simulink model "afe_abc_inv_3L_psm"  (R2025b)
settings: Solver=ode23tb  StartTime=0.0  StopTime=simlength  FixedStep=tc  MaxStep=tc
undefined symbols (not defined in the file or in its folder): Adrso, Amplitude_U, Amplitude_V, Amplitude_W, Aresd, b, Bresd, Cresd, Crso, CTRPIFF_CLIP_RELEASE, dead_time_AFE, dead_time_INV, deepNEGeta, deepNEGxi, deepPOSxi, emf_fb_p, emf_fb_p_ccaller_1, emf_fb_p_ccaller_2, emf_p, emf_p_ccaller_1, emf_p_ccaller_2, end_time_LVRT, fPWM_AFE, fPWM_INV, g0_161Hz, g0_500Hz, g1_161Hz, g1_500Hz, i_grid_neg_eta_lim, i_grid_neg_eta_red_lim, i_grid_neg_xi_lim, i_grid_neg_xi_red_lim, i_grid_pos_eta_lim, i_grid_pos_eta_red_lim, ibez, id_lim, ieta_neg_ref_lim, ieta_pos_ref_lim, Igrid_phase_normalization_factor, iq_lim, ixi_pos_ref_lim, Jm, k_frt_ref, kg, ki_afe, ki_i, ki_rc_neg_grid, ki_rc_pos_grid, ki_vs, ki_w, kp_afe, kp_i, kp_rc_neg_grid, kp_rc_pos_grid, kp_vs, kp_w, kw, l1, l2, Ld_norm ... (+48)
libraries: fl_lib x157, nesl_utility x86, cstblocks x14, simulink x13, single_phase_transformer_lib x3, threephase_inductor_lib x2, flexshaft_lib x1, pmsm_uvw_with_harmonics_lib x1
(part 6 of 11)

== system afe_abc_inv_3L_psm/afe_abc_inv_psm_mod1/inverter_control/current_ctrl/current_ctrl ==
  iq_ref : Inport
  MTPA : Subsystem
  Sqrt : Sqrt
  Square : Math  Operator=square
  Square1 : Math  Operator=square
  Sum : Sum  Inputs=|++
  To Workspace1 : ToWorkspace  VariableName=id_pu_sim  SampleTime=ts_inv
      settings: MaxDataPoints=Ns_inv
  To Workspace2 : ToWorkspace  VariableName=iq_pu_sim  SampleTime=ts_inv
      settings: MaxDataPoints=Ns_inv
  To Workspace3 : ToWorkspace  VariableName=id_ref_pu_sim  SampleTime=ts_inv
      settings: MaxDataPoints=Ns_inv
  To Workspace4 : ToWorkspace  VariableName=iq_ref_pu_sim  SampleTime=ts_inv
      settings: MaxDataPoints=Ns_inv
  To Workspace5 : ToWorkspace  VariableName=ud_pu_sim  SampleTime=ts_inv
      settings: MaxDataPoints=Ns_inv
  To Workspace6 : ToWorkspace  VariableName=uq_pu_sim  SampleTime=ts_inv
      settings: MaxDataPoints=Ns_inv
  To Workspace7 : ToWorkspace  VariableName=u_mot_pu_sim  SampleTime=ts_inv
      settings: MaxDataPoints=Ns_inv
  dq_pi_with_vector_antiwindup : Subsystem
  id_ref : Subsystem
      settings: PortSchema="{\"entries\":[{\"content\":{\"sides\":[{\"content\":{},\"type\":\"ConnectorPlacement.EquallySpacedRectSide\",\"uuid\":\"42af5d69-f0eb-42c6-9e03-28c1d0757323\"},{\"content\":{\"connectorIds\":[\"Out1\"],\"side\":\"RIGHT\"},\"type\":\"ConnectorPlacement.EquallySpacedRectSide\",\"uuid\":\"dd68a9f9-d15f-4e57-9d9e-130889a7b90c\"},{\"content\":{\"connectorIds\":[\"In1\"],\"side\":\"TOP\"},\"type\":\"ConnectorPlacement.EquallySpacedRectSide\",\"uuid\":\"68c797a2-8439-4b8d-8368-b7485adf0676\"}]},\"type\":\"ConnectorPlacement.EquallySpacedConnector\",\"uuid\":\"693c5f1c-0580-4626-8f13-b27865dfb3ac\"}],\"packageUris\":[\"http://schema.mathworks.com/mf0/Connector/R2020b\"],\"version\":\"1.0\"}"
  idref/id : Scope  NumInputPorts=2
      settings: SampleTime=tc  ActiveDisplayYMinimum=-0.65083541497562736  ActiveDisplayYMaximum=0.072495891063107235
  iqref/iq : Scope  NumInputPorts=2
      settings: SampleTime=tc  ActiveDisplayYMinimum=-1.1641617765003931  ActiveDisplayYMaximum=0.12935130850004364  DataLoggingVariableName=ScopeData2
  ud : Outport
  uq : Outport  Port=2
  tag scope: id_pu_ref=global, iq_pu_ref=global, u_mot_pu_sim=global, ud_pu_sim=global, uq_pu_sim=global
  wires:
  [iq_pu] -> To Workspace2/1, iqref/iq/2, dq_pi_with_vector_antiwindup/4(iq)  "iq"
  [id_pu] -> To Workspace1/1, idref/id/2, dq_pi_with_vector_antiwindup/2(id)  "id"
  MTPA/1(Id_ref_mtpa) -> id_ref/1(id_mtpa), [id_pu_ref]  "id_ref"
  iq_ref/1 -> MTPA/1(iq_ref), To Workspace4/1, iqref/iq/1, dq_pi_with_vector_antiwindup/3(iq_ref), [iq_pu_ref]  "iq_ref"
  dq_pi_with_vector_antiwindup/1(ctrl_d_u) -> To Workspace5/1, [ud_pu_sim], Square1/1, ud/1
  dq_pi_with_vector_antiwindup/2(ctrl_q_u) -> [uq_pu_sim], To Workspace6/1, Square/1, uq/1
  Square/1 -> Sum/1
  Sum/1 -> Sqrt/1
  Square1/1 -> Sum/2
  Sqrt/1 -> [u_mot_pu_sim], To Workspace7/1
  id_ref/1(id_ref) -> To Workspace3/1, dq_pi_with_vector_antiwindup/1(id_ref), idref/id/1  "id_ref"

== system afe_abc_inv_3L_psm/afe_abc_inv_psm_mod1/inverter_control/current_ctrl/current_transformation ==
  u : Inport
  v : Inport  Port=2
  w : Inport  Port=3
  To Workspace2 : ToWorkspace  VariableName=ialpha_pu_sim  SampleTime=ts_inv
      settings: MaxDataPoints=Ns_inv
  To Workspace3 : ToWorkspace  VariableName=ibeta_pu_sim  SampleTime=ts_inv
      settings: MaxDataPoints=Ns_inv
  alphabeta2dq : MATLAB Function  TreatAsAtomicUnit=on  SystemSampleTime=ts_inv
  uvw2alphabeta : MATLAB Function  TreatAsAtomicUnit=on  SystemSampleTime=ts_inv
  tag scope: ialpha_pu=global, ibeta_pu=global, id_pu=global, iq_pu=global
  wires:
  w/1 -> uvw2alphabeta/3(w)
  alphabeta2dq/2(q) -> [iq_pu]  "iq_pu"
  alphabeta2dq/1(d) -> [id_pu]  "id_pu"
  v/1 -> uvw2alphabeta/2(v)
  uvw2alphabeta/2(beta) -> To Workspace3/1, [ibeta_pu], alphabeta2dq/2(beta)  "ibeta_pu"
  uvw2alphabeta/1(alpha) -> To Workspace2/1, [ialpha_pu], alphabeta2dq/1(alpha)  "ialpha_pu"
  [theta_hat] -> alphabeta2dq/3(gamma)
  u/1 -> uvw2alphabeta/1(u)

== system afe_abc_inv_3L_psm/afe_abc_inv_psm_mod1/inverter_control/current_ctrl/sample_hold_normalization ==
  iu : Inport
  iv : Inport  Port=2
  iw : Inport  Port=3
  Gain : Gain  Gain=1/ibez
  Gain1 : Gain  Gain=1/ibez
  Gain2 : Gain  Gain=1/ibez
  Quantizer : Quantizer  QuantizationInterval=adc_quantization
  Quantizer1 : Quantizer  QuantizationInterval=adc_quantization
  Quantizer2 : Quantizer  QuantizationInterval=adc_quantization
  Unit Delay : UnitDelay  SampleTime=ts_inv  HasFrameUpgradeWarning=on
  Unit Delay1 : UnitDelay  SampleTime=ts_inv  HasFrameUpgradeWarning=on
  Unit Delay4 : UnitDelay  SampleTime=ts_inv  HasFrameUpgradeWarning=on
  Zero-Order Hold : ZeroOrderHold  SampleTime=ts_inv
  Zero-Order Hold1 : ZeroOrderHold  SampleTime=ts_inv
  Zero-Order Hold2 : ZeroOrderHold  SampleTime=ts_inv
  iu_pu : Outport
  iv_pu : Outport  Port=2
  iw_pu : Outport  Port=3
  wires:
  iu/1 -> Gain/1
  Zero-Order Hold1/1 -> Unit Delay1/1
  Zero-Order Hold2/1 -> Unit Delay4/1
  Zero-Order Hold/1 -> Unit Delay/1
  Unit Delay4/1 -> iw_pu/1
  Unit Delay1/1 -> iv_pu/1
  Unit Delay/1 -> iu_pu/1
  iw/1 -> Gain2/1
  iv/1 -> Gain1/1
  Gain2/1 -> Quantizer2/1
  Gain1/1 -> Quantizer1/1
  Gain/1 -> Quantizer/1
  Quantizer/1 -> Zero-Order Hold/1
  Quantizer1/1 -> Zero-Order Hold1/1
  Quantizer2/1 -> Zero-Order Hold2/1

== system afe_abc_inv_3L_psm/grid/grid_emulator/breaker/switch_1 ==
  Switch : fl_lib/Electrical/Electrical Elements/Switch  R_closed=Ron Ohm  G_open=1e-8 1/Ohm  Threshold=7.5  i_specify=off  i_priority=None  i=0 A  i_nominal_specify=off  i_nominal_value=1  i_nominal_unit=A  v_specify=off  v_priority=None  v=0 V  v_nominal_specify=off  v_nominal_value=1  v_nominal_unit=V
  snubber : fl_lib/Electrical/Electrical Elements/Capacitor  c=Csnubber F  r=Rsnubber Ohm  g=0 1/Ohm  i_specify=off  i_priority=None  i=0 A  i_nominal_specify=off  i_nominal_value=1  i_nominal_unit=A  v_specify=off  v_priority=None  v=0 V  v_nominal_specify=off  v_nominal_value=1  v_nominal_unit=V  vc_specify=off  vc_priority=High  vc=0 V  vc_nominal_specify=off  vc_nominal_value=1  vc_nominal_unit=V
  G : PMIOPort  Side=Left
  C : PMIOPort  Port=2  Side=Left
  E : PMIOPort  Port=3  Side=Right
  connections:
  Switch/RConn2 -- snubber/LConn1 -- C/RConn1
  Switch/RConn1 -- G/RConn1
  Switch/LConn1 -- snubber/RConn1 -- E/RConn1

== system afe_abc_inv_3L_psm/grid/grid_emulator/breaker/switch_2 ==
  Switch : fl_lib/Electrical/Electrical Elements/Switch  R_closed=Ron Ohm  G_open=1e-8 1/Ohm  Threshold=7.5  i_specify=off  i_priority=None  i=0 A  i_nominal_specify=off  i_nominal_value=1  i_nominal_unit=A  v_specify=off  v_priority=None  v=0 V  v_nominal_specify=off  v_nominal_value=1  v_nominal_unit=V
  snubber : fl_lib/Electrical/Electrical Elements/Capacitor  c=Csnubber F  r=Rsnubber Ohm  g=0 1/Ohm  i_specify=off  i_priority=None  i=0 A  i_nominal_specify=off  i_nominal_value=1  i_nominal_unit=A  v_specify=off  v_priority=None  v=0 V  v_nominal_specify=off  v_nominal_value=1  v_nominal_unit=V  vc_specify=off  vc_priority=High  vc=0 V  vc_nominal_specify=off  vc_nominal_value=1  vc_nominal_unit=V
  G : PMIOPort  Side=Left
  C : PMIOPort  Port=2  Side=Left
  E : PMIOPort  Port=3  Side=Right
  connections:
  snubber/RConn1 -- E/RConn1 -- Switch/LConn1
  Switch/RConn1 -- G/RConn1
  snubber/LConn1 -- C/RConn1 -- Switch/RConn2

== system afe_abc_inv_3L_psm/grid/grid_emulator/breaker/switch_3 ==
  Switch : fl_lib/Electrical/Electrical Elements/Switch  R_closed=Ron Ohm  G_open=1e-8 1/Ohm  Threshold=7.5  i_specify=off  i_priority=None  i=0 A  i_nominal_specify=off  i_nominal_value=1  i_nominal_unit=A  v_specify=off  v_priority=None  v=0 V  v_nominal_specify=off  v_nominal_value=1  v_nominal_unit=V
  snubber : fl_lib/Electrical/Electrical Elements/Capacitor  c=Csnubber F  r=Rsnubber Ohm  g=0 1/Ohm  i_specify=off  i_priority=None  i=0 A  i_nominal_specify=off  i_nominal_value=1  i_nominal_unit=A  v_specify=off  v_priority=None  v=0 V  v_nominal_specify=off  v_nominal_value=1  v_nominal_unit=V  vc_specify=off  vc_priority=High  vc=0 V  vc_nominal_specify=off  vc_nominal_value=1  vc_nominal_unit=V
  G : PMIOPort  Side=Left
  C : PMIOPort  Port=2  Side=Left
  E : PMIOPort  Port=3  Side=Right
  connections:
  Switch/RConn2 -- C/RConn1 -- snubber/LConn1
  Switch/RConn1 -- G/RConn1
  Switch/LConn1 -- E/RConn1 -- snubber/RConn1

== system afe_abc_inv_3L_psm/grid/grid_emulator/grid_emulator/phase_gen ==
  Constant4 : Constant  Value=omega_grid_emulator_nom
  Integrator : Integrator
  To Workspace7 : ToWorkspace  VariableName=gamma_grid_emulator_sim  SampleTime=ts_afe
      settings: MaxDataPoints=Ns_afe
  bounder1 : MATLAB Function  TreatAsAtomicUnit=on  SystemSampleTime=ts_afe
  grid_emu_phase : Outport  VectorParamsAs1DForOutWhenUnconnected=off
  tag scope: gamma_grid_emulator=global
  wires:
  bounder1/1(y) -> [gamma_grid_emulator], To Workspace7/1, grid_emu_phase/1  "grid_emu_phase"
  Constant4/1 -> Integrator/1
  Integrator/1 -> bounder1/1(u)

== system afe_abc_inv_3L_psm/grid/grid_emulator/grid_emulator/voltage_reference ==
  grid_emu_phase : Inport
  Vxi_p : Inport  Port=2
  Vxi_n : Inport  Port=3
  Veta_n : Inport  Port=4
  Constant2 : Constant  Value=0
  Sum1 : Sum  Inputs=|++
  Sum4 : Sum  Inputs=|++
  Variant Source : VariantSource  VariantControls={enable_frt_2 == 1, enable_frt_1 == 1}
  Variant Source1 : VariantSource  VariantControls={enable_frt_2 == 1, enable_frt_1 == 1}
  Variant Source2 : VariantSource  VariantControls={enable_frt_2 == 1, enable_frt_1 == 1}
  alphabeta2abc : MATLAB Function  TreatAsAtomicUnit=on  SystemSampleTime=ts_afe
  voltage_dource_with_frt : Subsystem
  xieta2alphabeta_neg : MATLAB Function  TreatAsAtomicUnit=on  SystemSampleTime=ts_afe
  xieta2alphabeta_pos : MATLAB Function  TreatAsAtomicUnit=on  SystemSampleTime=ts_afe
  V1_ref : Outport  VectorParamsAs1DForOutWhenUnconnected=off
  V2_ref : Outport  Port=2  VectorParamsAs1DForOutWhenUnconnected=off
  V3_ref : Outport  Port=3  VectorParamsAs1DForOutWhenUnconnected=off
  wires:
  xieta2alphabeta_pos/1(alpha) -> Sum1/1
  Sum1/1 -> alphabeta2abc/1(alpha)
  xieta2alphabeta_pos/2(beta) -> Sum4/1
  Sum4/1 -> alphabeta2abc/2(beta)
  xieta2alphabeta_neg/1(alpha) -> Sum1/2
  xieta2alphabeta_neg/2(beta) -> Sum4/2
  grid_emu_phase/1 -> voltage_dource_with_frt/1(gamma), xieta2alphabeta_neg/3(gamma), xieta2alphabeta_pos/3(gamma)
  Vxi_p/1 -> xieta2alphabeta_pos/1(xi)
  Constant2/1 -> xieta2alphabeta_pos/2(eta)
  Vxi_n/1 -> xieta2alphabeta_neg/1(xi)
  Veta_n/1 -> xieta2alphabeta_neg/2(eta)
  Variant Source/1 -> V1_ref/1
  alphabeta2abc/1(a) -> [V1_ref_xieta]
  alphabeta2abc/2(b) -> [V2_ref_xieta]
  alphabeta2abc/3(c) -> [V3_ref_xieta]
  voltage_dource_with_frt/3(vn_eta) -> [V3_ref_abc]
  voltage_dource_with_frt/2(vn_xi) -> [V2_ref_abc]
  voltage_dource_with_frt/1(vp_xi) -> [V1_ref_abc]
  [V1_ref_xieta] -> Variant Source/1
  [V1_ref_abc] -> Variant Source/2
  Variant Source1/1 -> V2_ref/1
  [V2_ref_xieta] -> Variant Source1/1
  [V2_ref_abc] -> Variant Source1/2
  Variant Source2/1 -> V3_ref/1
  [V3_ref_abc] -> Variant Source2/2
  [V3_ref_xieta] -> Variant Source2/1

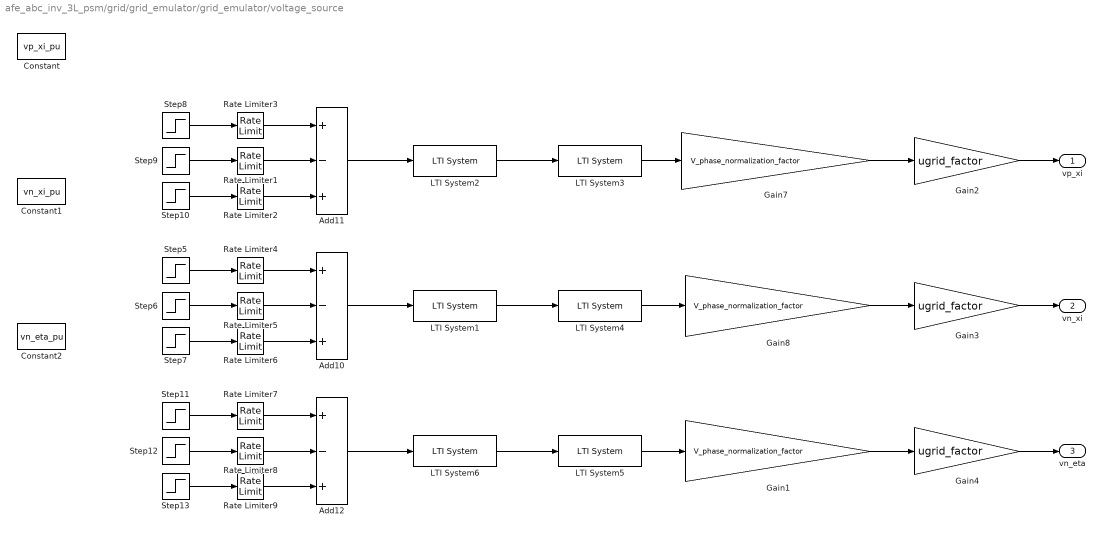
== system afe_abc_inv_3L_psm/grid/grid_emulator/grid_emulator/voltage_source ==
  Add10 : Sum  Inputs=+-+
  Add11 : Sum  Inputs=+-+
  Add12 : Sum  Inputs=+-+
  Constant : Constant  Value=vp_xi_pu
  Constant1 : Constant  Value=vn_xi_pu
  Constant2 : Constant  Value=vn_eta_pu
  Gain1 : Gain  Gain=V_phase_normalization_factor
  Gain2 : Gain  Gain=ugrid_factor
  Gain3 : Gain  Gain=ugrid_factor
  Gain4 : Gain  Gain=ugrid_factor
  Gain7 : Gain  Gain=V_phase_normalization_factor
  Gain8 : Gain  Gain=V_phase_normalization_factor
  LTI System1 : cstblocks/LTI System  sys=LVRT_flt_ss_c  IC=[0]  PadeOrder=0
  LTI System2 : cstblocks/LTI System  sys=LVRT_flt_ss_c  IC=[0]  PadeOrder=0
  LTI System3 : cstblocks/LTI System  sys=LVRT_flt_ss_c  IC=[]  PadeOrder=0
  LTI System4 : cstblocks/LTI System  sys=LVRT_flt_ss_c  IC=[]  PadeOrder=0
  LTI System5 : cstblocks/LTI System  sys=LVRT_flt_ss_c  IC=[]  PadeOrder=0
  LTI System6 : cstblocks/LTI System  sys=LVRT_flt_ss_c  IC=[0]  PadeOrder=0
  Rate Limiter{1..9} (9 alike) : RateLimiter  RisingSlewLimit=Vemu_ref_norm/t_ramp  FallingSlewLimit=-Vemu_ref_norm/t_ramp  SampleTimeMode=inherited
  Step10 : Step  Time=end_time_LVRT  After=vp_xi_pu*deepPOSxi  SampleTime=0
  Step11 : Step  Time=0  After=vn_eta_pu  SampleTime=0
  Step12 : Step  Time=start_time_LVRT  After=deepNEGeta  SampleTime=0
  Step13 : Step  Time=end_time_LVRT  After=deepNEGeta  SampleTime=0
  Step5 : Step  Time=0  After=vn_xi_pu  SampleTime=0
  Step6 : Step  Time=start_time_LVRT  After=deepNEGxi  SampleTime=0
  Step7 : Step  Time=end_time_LVRT  After=deepNEGxi  SampleTime=0
  Step8 : Step  Time=0  After=vp_xi_pu  SampleTime=0
  Step9 : Step  Time=start_time_LVRT  After=vp_xi_pu*deepPOSxi  SampleTime=0
  vp_xi : Outport  VectorParamsAs1DForOutWhenUnconnected=off
  vn_xi : Outport  Port=2  VectorParamsAs1DForOutWhenUnconnected=off
  vn_eta : Outport  Port=3  VectorParamsAs1DForOutWhenUnconnected=off
  wires:
  LTI System3/1 -> Gain7/1
  LTI System4/1 -> Gain8/1
  Gain7/1 -> Gain2/1
  Gain8/1 -> Gain3/1
  Gain1/1 -> Gain4/1
  LTI System5/1 -> Gain1/1
  Gain2/1 -> vp_xi/1
  Gain3/1 -> vn_xi/1
  Gain4/1 -> vn_eta/1
  LTI System6/1 -> LTI System5/1
  LTI System1/1 -> LTI System4/1
  LTI System2/1 -> LTI System3/1
  Rate Limiter2/1 -> Add11/3
  Add12/1 -> LTI System6/1
  Step7/1 -> Rate Limiter6/1
  Step6/1 -> Rate Limiter5/1
  Rate Limiter5/1 -> Add10/2
  Step5/1 -> Rate Limiter4/1
  Add11/1 -> LTI System2/1
  Rate Limiter7/1 -> Add12/1
  Step8/1 -> Rate Limiter3/1
  Step12/1 -> Rate Limiter8/1
  Step11/1 -> Rate Limiter7/1
  Rate Limiter1/1 -> Add11/2
  Step9/1 -> Rate Limiter1/1
  Rate Limiter3/1 -> Add11/1
  Rate Limiter8/1 -> Add12/2
  Rate Limiter9/1 -> Add12/3
  Rate Limiter4/1 -> Add10/1
  Rate Limiter6/1 -> Add10/3
  Step10/1 -> Rate Limiter2/1
  Add10/1 -> LTI System1/1
  Step13/1 -> Rate Limiter9/1

== system afe_abc_inv_3L_psm/grid/instantaneus_power/abc2alphabeta/abc2alphabeta ==
  a : Inport
  b : Inport  Port=2
  c : Inport  Port=3
  Gain1 : Gain  Gain=-1/2
  Gain11 : Gain  Gain=-1/2
  Gain2 : Gain  Gain=0
  Gain3 : Gain  Gain=sqrt(3)/2
  Gain4 : Gain  Gain=-sqrt(3)/2
  Gain8 : Gain  Gain=2/3
  Gain9 : Gain  Gain=2/3
  Sum : Sum  Inputs=+++
  Sum1 : Sum  Inputs=+++
  "alpha " : Outport  VectorParamsAs1DForOutWhenUnconnected=off
  "beta " : Outport  Port=2  VectorParamsAs1DForOutWhenUnconnected=off
  wires:
  Gain11/1 -> Sum/2
  Gain1/1 -> Sum/3
  Gain9/1 -> "beta "/1
  Gain8/1 -> "alpha "/1
  Gain2/1 -> Sum1/1
  Gain3/1 -> Sum1/2
  Gain4/1 -> Sum1/3
  a/1 -> Gain2/1, Sum/1
  c/1 -> Gain4/1, Gain1/1
  b/1 -> Gain3/1, Gain11/1
  Sum/1 -> Gain8/1
  Sum1/1 -> Gain9/1

== system afe_abc_inv_3L_psm/grid/instantaneus_power/abc2alphabeta /abc->alphabeta ==
  a : Inport
  b : Inport  Port=2
  c : Inport  Port=3
  Gain1 : Gain  Gain=-1/2
  Gain11 : Gain  Gain=-1/2
  Gain2 : Gain  Gain=0
  Gain3 : Gain  Gain=sqrt(3)/2
  Gain4 : Gain  Gain=-sqrt(3)/2
  Gain8 : Gain  Gain=2/3
  Gain9 : Gain  Gain=2/3
  Sum : Sum  Inputs=+++
  Sum1 : Sum  Inputs=+++
  "alpha " : Outport  VectorParamsAs1DForOutWhenUnconnected=off
  "beta " : Outport  Port=2  VectorParamsAs1DForOutWhenUnconnected=off
  wires:
  Sum1/1 -> Gain9/1
  Sum/1 -> Gain8/1
  b/1 -> Gain11/1, Gain3/1
  c/1 -> Gain1/1, Gain4/1
  a/1 -> Sum/1, Gain2/1
  Gain4/1 -> Sum1/3
  Gain3/1 -> Sum1/2
  Gain2/1 -> Sum1/1
  Gain8/1 -> "alpha "/1
  Gain9/1 -> "beta "/1
  Gain1/1 -> Sum/3
  Gain11/1 -> Sum/2

== system afe_abc_inv_3L_psm/afe_abc_inv_psm_mod1/afe/sv_pwm/modulator1/PWM generator u ==
  m : Inport
  phase : Inport  Port=2
  Bus Creator : BusCreator  Inputs=4
  Constant : Constant
  Gain : Gain  Gain=2
  Sum : Sum  Inputs=|+-
  carry_p : Subsystem
  modulator_n1 : Subsystem
  modulator_p1 : Subsystem
  mu : Outport
  wires:
  phase/1 -> carry_p/1(phase)
  carry_p/1(trp) -> modulator_n1/1(tr), modulator_p1/1(tr)  "trp"
  modulator_p1/1(m1) -> [m1]
  modulator_p1/2(m3) -> [m3]
  modulator_n1/1(m2) -> [m2]
  modulator_n1/2(m4) -> [m4]
  [m1] -> Bus Creator/1  "m1u"
  [m2] -> Bus Creator/2  "m2u"
  [m3] -> Bus Creator/3  "m3u"
  [m4] -> Bus Creator/4  "m4u"
  Bus Creator/1 -> mu/1  "p"
  m/1 -> Gain/1
  Gain/1 -> Sum/1
  Constant/1 -> Sum/2
  Sum/1 -> modulator_p1/2(m_index), modulator_n1/2(m_index)

== system afe_abc_inv_3L_psm/afe_abc_inv_psm_mod1/afe/sv_pwm/modulator1/PWM generator v ==
  m : Inport
  phase : Inport  Port=2
  Bus Creator : BusCreator  Inputs=4
  Constant : Constant
  Gain : Gain  Gain=2
  Sum : Sum  Inputs=|+-
  carry_p : Subsystem
  modulator_n1 : Subsystem
  modulator_p1 : Subsystem
  mv : Outport
  wires:
  Sum/1 -> modulator_n1/2(m_index), modulator_p1/2(m_index)
  Constant/1 -> Sum/2
  Gain/1 -> Sum/1
  m/1 -> Gain/1
  Bus Creator/1 -> mv/1  "p"
  [m4] -> Bus Creator/4  "m4v"
  [m3] -> Bus Creator/3  "m3v"
  [m2] -> Bus Creator/2  "m2v"
  [m1] -> Bus Creator/1  "m1v"
  modulator_n1/2(m4) -> [m4]
  modulator_n1/1(m2) -> [m2]
  modulator_p1/2(m3) -> [m3]
  modulator_p1/1(m1) -> [m1]
  carry_p/1(trp) -> modulator_p1/1(tr), modulator_n1/1(tr)  "trp"
  phase/1 -> carry_p/1(phase)

== system afe_abc_inv_3L_psm/afe_abc_inv_psm_mod1/afe/sv_pwm/modulator1/PWM generator w ==
  m : Inport
  phase : Inport  Port=2
  Bus Creator : BusCreator  Inputs=4
  Constant : Constant
  Gain : Gain  Gain=2
  Sum : Sum  Inputs=|+-
  carry_p : Subsystem
  modulator_n1 : Subsystem
  modulator_p1 : Subsystem
  mw : Outport
  wires:
  phase/1 -> carry_p/1(phase)
  carry_p/1(trp) -> modulator_n1/1(tr), modulator_p1/1(tr)  "trp"
  modulator_p1/1(m1) -> [m1]
  modulator_p1/2(m3) -> [m3]
  modulator_n1/1(m2) -> [m2]
  modulator_n1/2(m4) -> [m4]
  [m1] -> Bus Creator/1  "m1w"
  [m2] -> Bus Creator/2  "m2w"
  [m3] -> Bus Creator/3  "m3w"
  [m4] -> Bus Creator/4  "m4w"
  Bus Creator/1 -> mw/1  "p"
  m/1 -> Gain/1
  Gain/1 -> Sum/1
  Constant/1 -> Sum/2
  Sum/1 -> modulator_p1/2(m_index), modulator_n1/2(m_index)

== system afe_abc_inv_3L_psm/afe_abc_inv_psm_mod1/afe_control/current_ctrl/Inner Loop Current Control/Current-Control, Phase a ==
  In1 : Inport
  In2 : Inport  Port=2
  Add : Sum
  Cresd./Tcontrol new1 : Gain  Gain=Cresd  Multiplication=Matrix(K*u)
  Gain : Gain  Gain=kp_afe
  Gain1 : Gain  Gain=ki_afe
  Gain2 : Gain  Gain=Bresd  Multiplication=Matrix(K*u)
  Gain3 : Gain  Gain=Aresd  Multiplication=Matrix(K*u)
  Gain4 : Gain  Gain=1/ts_afe
  Gain5 : Gain  Gain=ts_afe
  Sum : Sum  Inputs=|+-
  Sum2 : Sum  Inputs=|++  SaturateOnIntegerOverflow=on
  Unit Delay : UnitDelay  InitialCondition=[0 0]  SampleTime=ts_afe  HasFrameUpgradeWarning=on
  Out1 : Outport
  wires:
  In1/1 -> Sum/1  "isa_ref"
  In2/1 -> Sum/2  "isa"
  Add/1 -> Out1/1  "v_a"
  Sum/1 -> Gain1/1, Gain/1
  Gain/1 -> Add/1
  Gain1/1 -> Gain2/1  "u(k)"
  Gain2/1 -> Gain5/1
  Gain5/1 -> Sum2/1
  Unit Delay/1 -> Gain3/1, Cresd./Tcontrol new1/1  "x(k)"
  Sum2/1 -> Unit Delay/1  "x(k+1)"
  Gain3/1 -> Sum2/2
  Cresd./Tcontrol new1/1 -> Gain4/1  "y(k)"
  Gain4/1 -> Add/2

== system afe_abc_inv_3L_psm/afe_abc_inv_psm_mod1/afe_control/current_ctrl/Inner Loop Current Control/Current-Control, Phase b ==
  In1 : Inport
  In2 : Inport  Port=2
  Add : Sum
  Cresd./Tcontrol new1 : Gain  Gain=Cresd  Multiplication=Matrix(K*u)
  Gain : Gain  Gain=kp_afe
  Gain1 : Gain  Gain=ki_afe
  Gain2 : Gain  Gain=Bresd  Multiplication=Matrix(K*u)
  Gain3 : Gain  Gain=Aresd  Multiplication=Matrix(K*u)
  Gain4 : Gain  Gain=1/ts_afe
  Gain5 : Gain  Gain=ts_afe
  Sum : Sum  Inputs=|+-
  Sum2 : Sum  Inputs=|++  SaturateOnIntegerOverflow=on
  Unit Delay : UnitDelay  InitialCondition=[0 0]  SampleTime=ts_afe  HasFrameUpgradeWarning=on
  Out1 : Outport
  wires:
  Cresd./Tcontrol new1/1 -> Gain4/1  "y(k)"
  Gain3/1 -> Sum2/2
  Sum2/1 -> Unit Delay/1  "x(k+1)"
  Unit Delay/1 -> Cresd./Tcontrol new1/1, Gain3/1  "x(k)"
  Gain5/1 -> Sum2/1
  Gain2/1 -> Gain5/1
  Gain1/1 -> Gain2/1  "u(k)"
  Gain/1 -> Add/1
  Sum/1 -> Gain/1, Gain1/1
  Add/1 -> Out1/1  "v_a"
  In2/1 -> Sum/2  "isb"
  In1/1 -> Sum/1  "isb_ref"
  Gain4/1 -> Add/2

== system afe_abc_inv_3L_psm/afe_abc_inv_psm_mod1/afe_control/current_ctrl/Inner Loop Current Control/Current-Control, Phase c ==
  In1 : Inport
  In2 : Inport  Port=2
  Add : Sum
  Cresd./Tcontrol new1 : Gain  Gain=Cresd  Multiplication=Matrix(K*u)
  Gain : Gain  Gain=kp_afe
  Gain1 : Gain  Gain=ki_afe
  Gain2 : Gain  Gain=Bresd  Multiplication=Matrix(K*u)
  Gain3 : Gain  Gain=Aresd  Multiplication=Matrix(K*u)
  Gain4 : Gain  Gain=1/ts_afe
  Gain5 : Gain  Gain=ts_afe
  Sum : Sum  Inputs=|+-
  Sum2 : Sum  Inputs=|++  SaturateOnIntegerOverflow=on
  Unit Delay : UnitDelay  InitialCondition=[0 0]  SampleTime=ts_afe  HasFrameUpgradeWarning=on
  Out1 : Outport
  wires:
  In1/1 -> Sum/1  "isc_ref"
  In2/1 -> Sum/2  "isc"
  Add/1 -> Out1/1  "v_a"
  Sum/1 -> Gain1/1, Gain/1
  Gain/1 -> Add/1
  Gain1/1 -> Gain2/1  "u(k)"
  Gain2/1 -> Gain5/1
  Gain5/1 -> Sum2/1
  Unit Delay/1 -> Gain3/1, Cresd./Tcontrol new1/1  "x(k)"
  Sum2/1 -> Unit Delay/1  "x(k+1)"
  Gain3/1 -> Sum2/2
  Cresd./Tcontrol new1/1 -> Gain4/1  "y(k)"
  Gain4/1 -> Add/2

== system afe_abc_inv_3L_psm/afe_abc_inv_psm_mod1/afe_control/current_sequence_avg/average_filter_ccaller/Moving Average Filter5 ==
  In2 : Inport
  In3 : Inport  Port=2
  Bus Selector : BusSelector  OutputSignals=ts,sshort,slong,pinput,cbpointer,cbsample,mavg_output
  C Caller : CCaller  FunctionName=mavgflt_process_simulink  PortSpecificationStruct="%)30     .    B H   8    (     @         %    \"     8    !     0         %  0 \"0    $    _    07)G3F%M90  4&]R=$YA;64 4V-O<&4     26YD97@     5'EP90      4VEZ90      27-';&]B86P   X    P    !@    @    $          4    (     0    ,    !         !   P!O=70 #@   #     &    \"     0         !0    @    !     P    $         $  # &]U=  .    .     8    (    !          %    \"     $    &     0         0   ...(+3251 chars)"  SampleTime=ts_afe
  Compare To Zero : simulink/Logic and Bit Operations/Compare To Zero  relop=>  OutDataTypeStr=boolean
  Constant : Constant  Value=5
  Constant5 : Constant  Value=ts_afe
  Data Type Conversion : DataTypeConversion  OutDataTypeStr=single  SaturateOnIntegerOverflow=off  RndMeth=Floor
  Data Type Conversion1 : DataTypeConversion  OutDataTypeStr=single  SaturateOnIntegerOverflow=off  RndMeth=Floor
  Data Type Conversion2 : DataTypeConversion  OutDataTypeStr=single  SaturateOnIntegerOverflow=off  RndMeth=Floor
  Data Type Conversion3 : DataTypeConversion  OutDataTypeStr=double  SaturateOnIntegerOverflow=off  RndMeth=Floor
  Data Type Conversion4 : DataTypeConversion  OutDataTypeStr=uint8  SaturateOnIntegerOverflow=off  RndMeth=Floor
  Data Type Conversion5 : DataTypeConversion  OutDataTypeStr=uint8  SaturateOnIntegerOverflow=off  RndMeth=Floor
  Enabled Subsystem : Subsystem  TreatAsAtomicUnit=on
  Reset Trigger : Subsystem
  Terminator{,1..5} (6 alike) : Terminator
  Zero-Order Hold1 : ZeroOrderHold  SampleTime=ts_afe
  Zero-Order Hold2 : ZeroOrderHold  SampleTime=ts_afe
  xi : Outport
  wires:
  Bus Selector/5 -> Terminator2/1  "<cbpointer>"
  Bus Selector/4 -> Terminator1/1  "<pinput>"
  Data Type Conversion3/1 -> xi/1  "output"
  Zero-Order Hold2/1 -> Data Type Conversion/1  "d1"
  Enabled Subsystem/1(Out1) -> Data Type Conversion1/1
  Compare To Zero/1 -> Enabled Subsystem/Enable
  In3/1 -> Enabled Subsystem/1(In1), Compare To Zero/1  "omega_grid"
  Constant5/1 -> Zero-Order Hold1/1
  Zero-Order Hold1/1 -> Data Type Conversion2/1  "d1"
  Bus Selector/3 -> Terminator4/1  "<slong>"
  Bus Selector/2 -> Terminator3/1  "<sshort>"
  Bus Selector/1 -> Terminator/1  "<ts>"
  C Caller/1 -> Bus Selector/1  "out"
  In2/1 -> Zero-Order Hold2/1  "input"
  Data Type Conversion4/1 -> C Caller/5
  Data Type Conversion/1 -> C Caller/1  "input"
  Data Type Conversion5/1 -> C Caller/4
  Data Type Conversion2/1 -> C Caller/3
  Data Type Conversion1/1 -> C Caller/2
  Reset Trigger/1(Out1) -> Data Type Conversion5/1
  Constant/1 -> Data Type Conversion4/1
  Bus Selector/6 -> Terminator5/1  "<cbsample>"
  Bus Selector/7 -> Data Type Conversion3/1  "<mavg_output>"

== system afe_abc_inv_3L_psm/afe_abc_inv_psm_mod1/afe_control/current_sequence_avg/average_filter_ccaller/Moving Average Filter6 ==
  In2 : Inport
  In3 : Inport  Port=2
  Bus Selector : BusSelector  OutputSignals=ts,sshort,slong,pinput,cbpointer,cbsample,mavg_output
  C Caller : CCaller  FunctionName=mavgflt_process_simulink  PortSpecificationStruct="%)30     .    B H   8    (     @         %    \"     8    !     0         %  0 \"0    $    _    07)G3F%M90  4&]R=$YA;64 4V-O<&4     26YD97@     5'EP90      4VEZ90      27-';&]B86P   X    P    !@    @    $          4    (     0    ,    !         !   P!O=70 #@   #     &    \"     0         !0    @    !     P    $         $  # &]U=  .    .     8    (    !          %    \"     $    &     0         0   ...(+3251 chars)"  SampleTime=ts_afe
  Compare To Zero : simulink/Logic and Bit Operations/Compare To Zero  relop=>  OutDataTypeStr=boolean
  Constant : Constant  Value=6
  Constant5 : Constant  Value=ts_afe
  Data Type Conversion : DataTypeConversion  OutDataTypeStr=single  SaturateOnIntegerOverflow=off  RndMeth=Floor
  Data Type Conversion1 : DataTypeConversion  OutDataTypeStr=single  SaturateOnIntegerOverflow=off  RndMeth=Floor
  Data Type Conversion2 : DataTypeConversion  OutDataTypeStr=single  SaturateOnIntegerOverflow=off  RndMeth=Floor
  Data Type Conversion3 : DataTypeConversion  OutDataTypeStr=double  SaturateOnIntegerOverflow=off  RndMeth=Floor
  Data Type Conversion4 : DataTypeConversion  OutDataTypeStr=uint8  SaturateOnIntegerOverflow=off  RndMeth=Floor
  Data Type Conversion5 : DataTypeConversion  OutDataTypeStr=uint8  SaturateOnIntegerOverflow=off  RndMeth=Floor
  Enabled Subsystem : Subsystem  TreatAsAtomicUnit=on
  Reset Trigger : Subsystem
  Terminator{,1..5} (6 alike) : Terminator
  Zero-Order Hold1 : ZeroOrderHold  SampleTime=ts_afe
  Zero-Order Hold2 : ZeroOrderHold  SampleTime=ts_afe
  xi : Outport
  wires:
  Bus Selector/7 -> Data Type Conversion3/1  "<mavg_output>"
  Bus Selector/6 -> Terminator5/1  "<cbsample>"
  Constant/1 -> Data Type Conversion4/1
  Reset Trigger/1(Out1) -> Data Type Conversion5/1
  Data Type Conversion1/1 -> C Caller/2
  Data Type Conversion2/1 -> C Caller/3
  Data Type Conversion5/1 -> C Caller/4
  Data Type Conversion/1 -> C Caller/1  "input"
  Data Type Conversion4/1 -> C Caller/5
  In2/1 -> Zero-Order Hold2/1  "input"
  C Caller/1 -> Bus Selector/1  "out"
  Bus Selector/1 -> Terminator/1  "<ts>"
  Bus Selector/2 -> Terminator3/1  "<sshort>"
  Bus Selector/3 -> Terminator4/1  "<slong>"
  Zero-Order Hold1/1 -> Data Type Conversion2/1  "d1"
  Constant5/1 -> Zero-Order Hold1/1
  In3/1 -> Compare To Zero/1, Enabled Subsystem/1(In1)  "omega_grid"
  Compare To Zero/1 -> Enabled Subsystem/Enable
  Enabled Subsystem/1(Out1) -> Data Type Conversion1/1
  Zero-Order Hold2/1 -> Data Type Conversion/1  "d1"
  Data Type Conversion3/1 -> xi/1  "output"
  Bus Selector/4 -> Terminator1/1  "<pinput>"
  Bus Selector/5 -> Terminator2/1  "<cbpointer>"

== system afe_abc_inv_3L_psm/afe_abc_inv_psm_mod1/afe_control/current_sequence_avg/average_filter_ccaller/Moving Average Filter7 ==
  In2 : Inport
  In3 : Inport  Port=2
  Bus Selector : BusSelector  OutputSignals=ts,sshort,slong,pinput,cbpointer,cbsample,mavg_output
  C Caller : CCaller  FunctionName=mavgflt_process_simulink  PortSpecificationStruct="%)30     .    B H   8    (     @         %    \"     8    !     0         %  0 \"0    $    _    07)G3F%M90  4&]R=$YA;64 4V-O<&4     26YD97@     5'EP90      4VEZ90      27-';&]B86P   X    P    !@    @    $          4    (     0    ,    !         !   P!O=70 #@   #     &    \"     0         !0    @    !     P    $         $  # &]U=  .    .     8    (    !          %    \"     $    &     0         0   ...(+3251 chars)"  SampleTime=ts_afe
  Compare To Zero : simulink/Logic and Bit Operations/Compare To Zero  relop=>  OutDataTypeStr=boolean
  Constant : Constant  Value=7
  Constant5 : Constant  Value=ts_afe
  Data Type Conversion : DataTypeConversion  OutDataTypeStr=single  SaturateOnIntegerOverflow=off  RndMeth=Floor
  Data Type Conversion1 : DataTypeConversion  OutDataTypeStr=single  SaturateOnIntegerOverflow=off  RndMeth=Floor
  Data Type Conversion2 : DataTypeConversion  OutDataTypeStr=single  SaturateOnIntegerOverflow=off  RndMeth=Floor
  Data Type Conversion3 : DataTypeConversion  OutDataTypeStr=double  SaturateOnIntegerOverflow=off  RndMeth=Floor
  Data Type Conversion4 : DataTypeConversion  OutDataTypeStr=uint8  SaturateOnIntegerOverflow=off  RndMeth=Floor
  Data Type Conversion5 : DataTypeConversion  OutDataTypeStr=uint8  SaturateOnIntegerOverflow=off  RndMeth=Floor
  Enabled Subsystem : Subsystem  TreatAsAtomicUnit=on
  Reset Trigger : Subsystem
  Terminator{,1..5} (6 alike) : Terminator
  Zero-Order Hold1 : ZeroOrderHold  SampleTime=ts_afe
  Zero-Order Hold2 : ZeroOrderHold  SampleTime=ts_afe
  xi : Outport
  wires:
  Bus Selector/5 -> Terminator2/1  "<cbpointer>"
  Bus Selector/4 -> Terminator1/1  "<pinput>"
  Data Type Conversion3/1 -> xi/1  "output"
  Zero-Order Hold2/1 -> Data Type Conversion/1  "d1"
  Enabled Subsystem/1(Out1) -> Data Type Conversion1/1
  Compare To Zero/1 -> Enabled Subsystem/Enable
  In3/1 -> Enabled Subsystem/1(In1), Compare To Zero/1  "omega_grid"
  Constant5/1 -> Zero-Order Hold1/1
  Zero-Order Hold1/1 -> Data Type Conversion2/1  "d1"
  Bus Selector/3 -> Terminator4/1  "<slong>"
  Bus Selector/2 -> Terminator3/1  "<sshort>"
  Bus Selector/1 -> Terminator/1  "<ts>"
  C Caller/1 -> Bus Selector/1  "out"
  In2/1 -> Zero-Order Hold2/1  "input"
  Data Type Conversion4/1 -> C Caller/5
  Data Type Conversion/1 -> C Caller/1  "input"
  Data Type Conversion5/1 -> C Caller/4
  Data Type Conversion2/1 -> C Caller/3
  Data Type Conversion1/1 -> C Caller/2
  Reset Trigger/1(Out1) -> Data Type Conversion5/1
  Constant/1 -> Data Type Conversion4/1
  Bus Selector/6 -> Terminator5/1  "<cbsample>"
  Bus Selector/7 -> Data Type Conversion3/1  "<mavg_output>"

== system afe_abc_inv_3L_psm/afe_abc_inv_psm_mod1/afe_control/current_sequence_avg/average_filter_ccaller/Moving Average Filter8 ==
  In2 : Inport
  In3 : Inport  Port=2
  Bus Selector : BusSelector  OutputSignals=ts,sshort,slong,pinput,cbpointer,cbsample,mavg_output
  C Caller : CCaller  FunctionName=mavgflt_process_simulink  PortSpecificationStruct="%)30     .    B H   8    (     @         %    \"     8    !     0         %  0 \"0    $    _    07)G3F%M90  4&]R=$YA;64 4V-O<&4     26YD97@     5'EP90      4VEZ90      27-';&]B86P   X    P    !@    @    $          4    (     0    ,    !         !   P!O=70 #@   #     &    \"     0         !0    @    !     P    $         $  # &]U=  .    .     8    (    !          %    \"     $    &     0         0   ...(+3251 chars)"  SampleTime=ts_afe
  Compare To Zero : simulink/Logic and Bit Operations/Compare To Zero  relop=>  OutDataTypeStr=boolean
  Constant : Constant  Value=8
  Constant5 : Constant  Value=ts_afe
  Data Type Conversion : DataTypeConversion  OutDataTypeStr=single  SaturateOnIntegerOverflow=off  RndMeth=Floor
  Data Type Conversion1 : DataTypeConversion  OutDataTypeStr=single  SaturateOnIntegerOverflow=off  RndMeth=Floor
  Data Type Conversion2 : DataTypeConversion  OutDataTypeStr=single  SaturateOnIntegerOverflow=off  RndMeth=Floor
  Data Type Conversion3 : DataTypeConversion  OutDataTypeStr=double  SaturateOnIntegerOverflow=off  RndMeth=Floor
  Data Type Conversion4 : DataTypeConversion  OutDataTypeStr=uint8  SaturateOnIntegerOverflow=off  RndMeth=Floor
  Data Type Conversion5 : DataTypeConversion  OutDataTypeStr=uint8  SaturateOnIntegerOverflow=off  RndMeth=Floor
  Enabled Subsystem : Subsystem  TreatAsAtomicUnit=on
  Reset Trigger : Subsystem
  Terminator{,1..5} (6 alike) : Terminator
  Zero-Order Hold1 : ZeroOrderHold  SampleTime=ts_afe
  Zero-Order Hold2 : ZeroOrderHold  SampleTime=ts_afe
  xi : Outport
  wires:
  Bus Selector/7 -> Data Type Conversion3/1  "<mavg_output>"
  Bus Selector/6 -> Terminator5/1  "<cbsample>"
  Constant/1 -> Data Type Conversion4/1
  Reset Trigger/1(Out1) -> Data Type Conversion5/1
  Data Type Conversion1/1 -> C Caller/2
  Data Type Conversion2/1 -> C Caller/3
  Data Type Conversion5/1 -> C Caller/4
  Data Type Conversion/1 -> C Caller/1  "input"
  Data Type Conversion4/1 -> C Caller/5
  In2/1 -> Zero-Order Hold2/1  "input"
  C Caller/1 -> Bus Selector/1  "out"
  Bus Selector/1 -> Terminator/1  "<ts>"
  Bus Selector/2 -> Terminator3/1  "<sshort>"
  Bus Selector/3 -> Terminator4/1  "<slong>"
  Zero-Order Hold1/1 -> Data Type Conversion2/1  "d1"
  Constant5/1 -> Zero-Order Hold1/1
  In3/1 -> Compare To Zero/1, Enabled Subsystem/1(In1)  "omega_grid"
  Compare To Zero/1 -> Enabled Subsystem/Enable
  Enabled Subsystem/1(Out1) -> Data Type Conversion1/1
  Zero-Order Hold2/1 -> Data Type Conversion/1  "d1"
  Data Type Conversion3/1 -> xi/1  "output"
  Bus Selector/4 -> Terminator1/1  "<pinput>"
  Bus Selector/5 -> Terminator2/1  "<cbpointer>"

== system afe_abc_inv_3L_psm/afe_abc_inv_psm_mod1/afe_control/current_sequence_avg/average_filter_simulink/mavg_1 ==
  in : Inport
  Gain : Gain  Gain=n1-1
  Gain1 : Gain  Gain=1/n1
  Sum : Sum  Inputs=|++
  Unit Delay : UnitDelay  SampleTime=ts_afe  HasFrameUpgradeWarning=on
  out : Outport  VectorParamsAs1DForOutWhenUnconnected=off
  wires:
  Sum/1 -> Gain1/1
  Unit Delay/1 -> Gain/1
  in/1 -> Sum/1
  Gain1/1 -> out/1, Unit Delay/1
  Gain/1 -> Sum/2

== system afe_abc_inv_3L_psm/afe_abc_inv_psm_mod1/afe_control/current_sequence_avg/average_filter_simulink/mavg_2 ==
  in : Inport
  Gain : Gain  Gain=n1-1
  Gain1 : Gain  Gain=1/n1
  Sum : Sum  Inputs=|++
  Unit Delay : UnitDelay  SampleTime=ts_afe  HasFrameUpgradeWarning=on
  out : Outport  VectorParamsAs1DForOutWhenUnconnected=off
  wires:
  Gain/1 -> Sum/2
  Gain1/1 -> Unit Delay/1, out/1
  in/1 -> Sum/1
  Unit Delay/1 -> Gain/1
  Sum/1 -> Gain1/1

== system afe_abc_inv_3L_psm/afe_abc_inv_psm_mod1/afe_control/current_sequence_avg/average_filter_simulink/mavg_3 ==
  in : Inport
  Gain : Gain  Gain=n1-1
  Gain1 : Gain  Gain=1/n1
  Sum : Sum  Inputs=|++
  Unit Delay : UnitDelay  SampleTime=ts_afe  HasFrameUpgradeWarning=on
  out : Outport  VectorParamsAs1DForOutWhenUnconnected=off
  wires:
  Sum/1 -> Gain1/1
  Unit Delay/1 -> Gain/1
  in/1 -> Sum/1
  Gain1/1 -> out/1, Unit Delay/1
  Gain/1 -> Sum/2

== system afe_abc_inv_3L_psm/afe_abc_inv_psm_mod1/afe_control/current_sequence_avg/average_filter_simulink/mavg_4 ==
  in : Inport
  Gain : Gain  Gain=n1-1
  Gain1 : Gain  Gain=1/n1
  Sum : Sum  Inputs=|++
  Unit Delay : UnitDelay  SampleTime=ts_afe  HasFrameUpgradeWarning=on
  out : Outport  VectorParamsAs1DForOutWhenUnconnected=off
  wires:
  Gain/1 -> Sum/2
  Gain1/1 -> Unit Delay/1, out/1
  in/1 -> Sum/1
  Unit Delay/1 -> Gain/1
  Sum/1 -> Gain1/1
